simulink model "SchultzExample"  (R2017b)
settings: Solver=ode3  StartTime=0.0  StopTime=10.0  FixedStep=Ts  RelTol=1e-3
PreLoadFcn:
  | waijung.modelPreload; % Required for working with Waijung Blockset. Do not remove.
undefined symbols (not defined in the file): FiO2, HCLK, HSEOSC, Link, LQFP100, ST, STM32F407VG, STM32F4DISCOVERY, Ts
libraries: stm32f4_i2c_lib x17, simulink x3, stm32f4_io_lib x1, stm32f4_device_config_lib x1
(part 2 of 2)

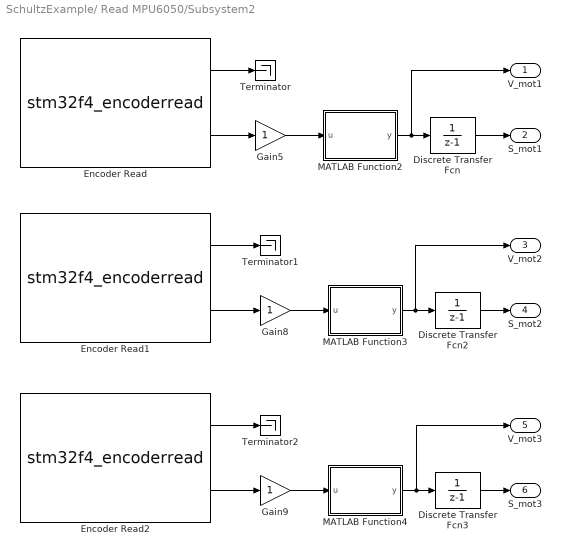
== system SchultzExample/ Read MPU6050/Subsystem2 ==
  Discrete Transfer Fcn : DiscreteTransferFcn  Denominator=[1 -1]
  Discrete Transfer Fcn2 : DiscreteTransferFcn  Denominator=[1 -1]
  Discrete Transfer Fcn3 : DiscreteTransferFcn  Denominator=[1 -1]
  Encoder Read : S-Function  FunctionName=stm32f4_encoderread  Parameters=sampletime,sampletimestr,blockid,timer,apb,portstr,pinstr,pinmat,chmat,filterstr,filter,factor,rstcnt,ppr  SFunctionDeploymentMode=off  EnableBusSupport=off  mask(stm32f4_encoderread){timer=3, ch1=B4, ch2=B5, ppr=65536, rstcnt=on, filterstr=No filter; sampling is done at fDTS, sampletime=Ts, sampletimestr=-1, blockid=ReadMPU6050Subsystem2EncoderRead, absresetinput=off, portpinstr=B4,B5, portstr=["B"], pinstr=["GPIO_Pin_4 | GPIO_Pin_5"], pinmat=[2 4 5], chmat=[1  2], apb=1, filter=0, factor=4}
      mask prompts: ch1 "Channel A Input Pin"; ch2 "Channel B Input Pin"; ppr "PPR (Number of pulses generated per revolution)"; rstcnt "Reset counter after every counter read"; filterstr "Built-in Input Capture Filter"; sampletime "Sample time (sec)"; sampletimestr "Compiled sample time (sec) in string"; absresetinput "Enable absolute position reset input signal"; portpinstr "Port pin string"; portstr "Port string"; pinstr "Pin string"; pinmat "Pin matrix"; chmat "Channel order"; filter "Filter ID"
      mask help:
      | The output Direction (uint32) is the direction of rotation either 0 or 1.
      |
      | The output Position (count) (uint32) is the count of number of edges of the encoder output signals from either channel A and B. The decoder is set to count at every rising and falling edge of both channel A and B (4x) or (x2) for one channel. For example, if an encoder has 180 pulses per revolution (PPS) and two channels are selected, the maximum count is 720 per revolution (4x180 = 720), i.e. from 0 to 719.
      mask init:
      | stm32f4_encoderread_callback('init');
      mask Help: web(fullfile(waijungdocroot,'stm32f4_encoderread.htm'),'-browser')
      mask TypeOptions timer: 1 | 2 | 3 | 4 | 5 | 8
      mask Callback timer: stm32f4_encoderread_callback('timer');
      mask TypeOptions ch1: Not available - Do not use | A6 | C6 | B4
      mask Callback ch1: stm32f4_encoderread_callback('chA');
      mask TypeOptions ch2: Not available - Do not use | A7 | C7 | B5
      mask Callback ch2: stm32f4_encoderread_callback('chB');
      mask Callback ppr: stm32f4_encoderread_callback('ppr');
      mask Callback rstcnt: stm32f4_encoderread_callback('rstcnt');
      mask TypeOptions filterstr: No filter; sampling is done at fDTS | fSAMPLING=fCK_INT; N=2 | fSAMPLING=fCK_INT; N=4 | fSAMPLING=fCK_INT; N=8 | fSAMPLING=fDTS/2; N=6 | fSAMPLING=fDTS/2; N=8 | fSAMPLING=fDTS/4; N=6 | fSAMPLING=fDTS/4; N=8 | fSAMPLING=fDTS/8; N=6 | fSAMPLING=fDTS/8; N=8 | fSAMPLING=fDTS/16; N=5 | fSAMPLING=fDTS/16; N=6 | fSAMPLING=fDTS/16; N=8 | fSAMPLING=fDTS/32; N=5 | fSAMPLING=fDTS/32; N=6 | fSAMPLING=fDTS/32; N=8
      mask Callback filterstr: stm32f4_encoderread_callback('filterstr');
      mask Callback sampletimestr: stm32f4_encoderread_callback('sampletimestr');
      mask Callback blockid: stm32f4_encoderread_callback('blockid');
      mask Display: text(0.05, 0.5, 'Timer: 3\nInput pins [CH_A, CH_B]: [B4,B5]\nRST Counter: Yes\nTs (sec): -1','ver','middle','hor','left');port_label('output', 1, 'Direction');port_label('output', 2, 'Position (count)')
  Encoder Read1 : S-Function  FunctionName=stm32f4_encoderread  Parameters=sampletime,sampletimestr,blockid,timer,apb,portstr,pinstr,pinmat,chmat,filterstr,filter,factor,rstcnt,ppr  SFunctionDeploymentMode=off  EnableBusSupport=off  mask(stm32f4_encoderread){timer=1, ch1=E9, ch2=E11, ppr=65536, rstcnt=on, filterstr=No filter; sampling is done at fDTS, sampletime=Ts, sampletimestr=-1, blockid=ReadMPU6050Subsystem2EncoderRead1, absresetinput=off, portpinstr=E9,E11, portstr=["E"], pinstr=["GPIO_Pin_9 | GPIO_Pin_11"], pinmat=[2 9 11], chmat=[1  2], apb=2, filter=0, factor=4}
      mask prompts: ch1 "Channel A Input Pin"; ch2 "Channel B Input Pin"; ppr "PPR (Number of pulses generated per revolution)"; rstcnt "Reset counter after every counter read"; filterstr "Built-in Input Capture Filter"; sampletime "Sample time (sec)"; sampletimestr "Compiled sample time (sec) in string"; absresetinput "Enable absolute position reset input signal"; portpinstr "Port pin string"; portstr "Port string"; pinstr "Pin string"; pinmat "Pin matrix"; chmat "Channel order"; filter "Filter ID"
      mask help:
      | The output Direction (uint32) is the direction of rotation either 0 or 1.
      |
      | The output Position (count) (uint32) is the count of number of edges of the encoder output signals from either channel A and B. The decoder is set to count at every rising and falling edge of both channel A and B (4x) or (x2) for one channel. For example, if an encoder has 180 pulses per revolution (PPS) and two channels are selected, the maximum count is 720 per revolution (4x180 = 720), i.e. from 0 to 719.
      mask init:
      | stm32f4_encoderread_callback('init');
      mask Help: web(fullfile(waijungdocroot,'stm32f4_encoderread.htm'),'-browser')
      mask TypeOptions timer: 1 | 2 | 3 | 4 | 5 | 8
      mask Callback timer: stm32f4_encoderread_callback('timer');
      mask TypeOptions ch1: Not available - Do not use | E9 | A8
      mask Callback ch1: stm32f4_encoderread_callback('chA');
      mask TypeOptions ch2: Not available - Do not use | E11 | A9
      mask Callback ch2: stm32f4_encoderread_callback('chB');
      mask Callback ppr: stm32f4_encoderread_callback('ppr');
      mask Callback rstcnt: stm32f4_encoderread_callback('rstcnt');
      mask TypeOptions filterstr: No filter; sampling is done at fDTS | fSAMPLING=fCK_INT; N=2 | fSAMPLING=fCK_INT; N=4 | fSAMPLING=fCK_INT; N=8 | fSAMPLING=fDTS/2; N=6 | fSAMPLING=fDTS/2; N=8 | fSAMPLING=fDTS/4; N=6 | fSAMPLING=fDTS/4; N=8 | fSAMPLING=fDTS/8; N=6 | fSAMPLING=fDTS/8; N=8 | fSAMPLING=fDTS/16; N=5 | fSAMPLING=fDTS/16; N=6 | fSAMPLING=fDTS/16; N=8 | fSAMPLING=fDTS/32; N=5 | fSAMPLING=fDTS/32; N=6 | fSAMPLING=fDTS/32; N=8
      mask Callback filterstr: stm32f4_encoderread_callback('filterstr');
      mask Callback sampletimestr: stm32f4_encoderread_callback('sampletimestr');
      mask Callback blockid: stm32f4_encoderread_callback('blockid');
      mask Display: text(0.05, 0.5, 'Timer: 1\nInput pins [CH_A, CH_B]: [E9,E11]\nRST Counter: Yes\nTs (sec): -1','ver','middle','hor','left');port_label('output', 1, 'Direction');port_label('output', 2, 'Position (count)')
  Encoder Read2 : S-Function  FunctionName=stm32f4_encoderread  Parameters=sampletime,sampletimestr,blockid,timer,apb,portstr,pinstr,pinmat,chmat,filterstr,filter,factor,rstcnt,ppr  SFunctionDeploymentMode=off  EnableBusSupport=off  mask(stm32f4_encoderread){timer=8, ch1=C6, ch2=C7, ppr=65536, rstcnt=on, filterstr=No filter; sampling is done at fDTS, sampletime=Ts, sampletimestr=-1, blockid=ReadMPU6050Subsystem2EncoderRead2, absresetinput=off, portpinstr=C6,C7, portstr=["C"], pinstr=["GPIO_Pin_6 | GPIO_Pin_7"], pinmat=[2 6 7], chmat=[1  2], apb=2, filter=0, factor=4}
      mask prompts: ch1 "Channel A Input Pin"; ch2 "Channel B Input Pin"; ppr "PPR (Number of pulses generated per revolution)"; rstcnt "Reset counter after every counter read"; filterstr "Built-in Input Capture Filter"; sampletime "Sample time (sec)"; sampletimestr "Compiled sample time (sec) in string"; absresetinput "Enable absolute position reset input signal"; portpinstr "Port pin string"; portstr "Port string"; pinstr "Pin string"; pinmat "Pin matrix"; chmat "Channel order"; filter "Filter ID"
      mask help:
      | The output Direction (uint32) is the direction of rotation either 0 or 1.
      |
      | The output Position (count) (uint32) is the count of number of edges of the encoder output signals from either channel A and B. The decoder is set to count at every rising and falling edge of both channel A and B (4x) or (x2) for one channel. For example, if an encoder has 180 pulses per revolution (PPS) and two channels are selected, the maximum count is 720 per revolution (4x180 = 720), i.e. from 0 to 719.
      mask init:
      | stm32f4_encoderread_callback('init');
      mask Help: web(fullfile(waijungdocroot,'stm32f4_encoderread.htm'),'-browser')
      mask TypeOptions timer: 1 | 2 | 3 | 4 | 5 | 8
      mask Callback timer: stm32f4_encoderread_callback('timer');
      mask TypeOptions ch1: Not available - Do not use | A6 | C6 | B4
      mask Callback ch1: stm32f4_encoderread_callback('chA');
      mask TypeOptions ch2: Not available - Do not use | A7 | C7 | B5
      mask Callback ch2: stm32f4_encoderread_callback('chB');
      mask Callback ppr: stm32f4_encoderread_callback('ppr');
      mask Callback rstcnt: stm32f4_encoderread_callback('rstcnt');
      mask TypeOptions filterstr: No filter; sampling is done at fDTS | fSAMPLING=fCK_INT; N=2 | fSAMPLING=fCK_INT; N=4 | fSAMPLING=fCK_INT; N=8 | fSAMPLING=fDTS/2; N=6 | fSAMPLING=fDTS/2; N=8 | fSAMPLING=fDTS/4; N=6 | fSAMPLING=fDTS/4; N=8 | fSAMPLING=fDTS/8; N=6 | fSAMPLING=fDTS/8; N=8 | fSAMPLING=fDTS/16; N=5 | fSAMPLING=fDTS/16; N=6 | fSAMPLING=fDTS/16; N=8 | fSAMPLING=fDTS/32; N=5 | fSAMPLING=fDTS/32; N=6 | fSAMPLING=fDTS/32; N=8
      mask Callback filterstr: stm32f4_encoderread_callback('filterstr');
      mask Callback sampletimestr: stm32f4_encoderread_callback('sampletimestr');
      mask Callback blockid: stm32f4_encoderread_callback('blockid');
      mask Display: text(0.05, 0.5, 'Timer: 8\nInput pins [CH_A, CH_B]: [C6,C7]\nRST Counter: Yes\nTs (sec): -1','ver','middle','hor','left');port_label('output', 1, 'Direction');port_label('output', 2, 'Position (count)')
  Gain5 : Gain  OutDataTypeStr=double
  Gain8 : Gain  OutDataTypeStr=double
  Gain9 : Gain  OutDataTypeStr=double
  MATLAB Function2 : MATLAB Function  TreatAsAtomicUnit=on
  MATLAB Function3 : MATLAB Function  TreatAsAtomicUnit=on
  MATLAB Function4 : MATLAB Function  TreatAsAtomicUnit=on
  Terminator : Terminator
  Terminator1 : Terminator
  Terminator2 : Terminator
  V_mot1 : Outport
  S_mot1 : Outport  Port=2
  V_mot2 : Outport  Port=3
  S_mot2 : Outport  Port=4
  V_mot3 : Outport  Port=5
  S_mot3 : Outport  Port=6
  wires:
  Encoder Read2/1 -> Terminator2/1
  Encoder Read1/1 -> Terminator1/1
  Encoder Read/1 -> Terminator/1
  Discrete Transfer Fcn/1 -> S_mot1/1
  Discrete Transfer Fcn2/1 -> S_mot2/1
  Discrete Transfer Fcn3/1 -> S_mot3/1
  Encoder Read2/2 -> Gain9/1
  MATLAB Function4/1(y) -> Discrete Transfer Fcn3/1, V_mot3/1
  Gain9/1 -> MATLAB Function4/1(u)
  Encoder Read1/2 -> Gain8/1
  MATLAB Function3/1(y) -> Discrete Transfer Fcn2/1, V_mot2/1
  Gain8/1 -> MATLAB Function3/1(u)
  MATLAB Function2/1(y) -> Discrete Transfer Fcn/1, V_mot1/1
  Encoder Read/2 -> Gain5/1
  Gain5/1 -> MATLAB Function2/1(u)

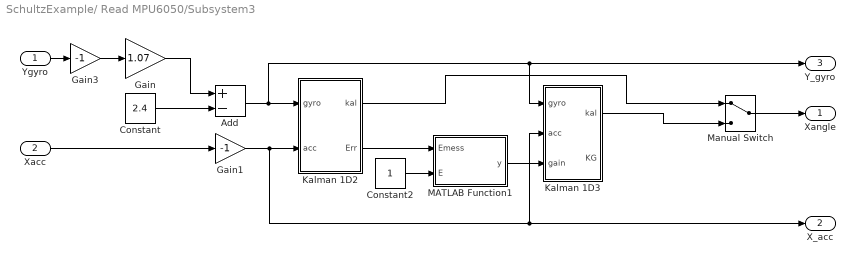
== system SchultzExample/ Read MPU6050/Subsystem3 ==
  Ygyro : Inport
  Xacc : Inport  Port=2
  Add : Sum  Inputs=+-
  Constant : Constant  Value=2.4
  Constant2 : Constant
  Gain : Gain  Gain=1.07
  Gain1 : Gain  Gain=-1  OutDataTypeStr=double
  Gain3 : Gain  Gain=-1  OutDataTypeStr=double
  Kalman 1D2 : Subsystem
  Kalman 1D3 : Subsystem
  MATLAB Function1 : MATLAB Function  TreatAsAtomicUnit=on
  Manual Switch : ManualSwitch
  Xangle : Outport
  X_acc : Outport  Port=2
  Y_gyro : Outport  Port=3
  wires:
  Constant/1 -> Add/2
  Gain/1 -> Add/1
  Gain3/1 -> Gain/1
  Add/1 -> Kalman 1D2/1(gyro), Y_gyro/1, Kalman 1D3/1(gyro)
  Gain1/1 -> Kalman 1D2/2(acc), Kalman 1D3/2(acc), X_acc/1
  MATLAB Function1/1(y) -> Kalman 1D3/3(gain)
  Kalman 1D2/2(Err) -> MATLAB Function1/1(Emess)
  Constant2/1 -> MATLAB Function1/2(E)
  Xacc/1 -> Gain1/1
  Ygyro/1 -> Gain3/1
  Manual Switch/1 -> Xangle/1
  Kalman 1D2/1(kal) -> Manual Switch/1
  Kalman 1D3/1(kal) -> Manual Switch/2

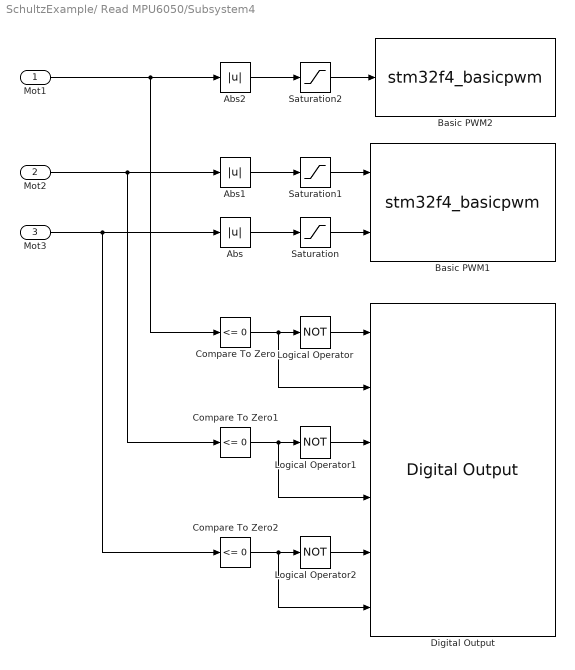
== system SchultzExample/ Read MPU6050/Subsystem4 ==
  Mot1 : Inport
  Mot2 : Inport  Port=2
  Mot3 : Inport  Port=3
  Abs : Abs
  Abs1 : Abs
  Abs2 : Abs
  Basic PWM1 : S-Function  FunctionName=stm32f4_basicpwm  Parameters=timer,pwmperiod,ch1pin,ch2pin,ch3pin,ch4pin,sampletime,sampletimestr,blockid,apb,portstr,pinstr,pinmat,timarr,timprescale,chmat,polaritystr  SFunctionDeploymentMode=off  EnableBusSupport=off  mask(stm32f4_basicpwm){timer=9, pwmperiod=50e-6, polarity=Active High, polaritystr=TIM_OCPolarity_High, ch1pin=A2, ch2pin=E6, ch3pin=Not available - Do not use, ch4pin=Not available - Do not use, sampletime=Ts, sampletimestr=-1, blockid=ReadMPU6050Subsystem4BasicPWM1, portpinstr=A2,E6,,, enablecustomportlabel=off, cinputportlabel=In1, In2, In3, In4, coutputportlabel=0, apb=2, portstr=["A","E"], pinstr=["GPIO_Pin_2","GPIO_Pin_6"], pinmat=[1 2;1 6], timarr=8399, timprescale=0, chmat=[1  2]}
      mask prompts: pwmperiod "PWM Period (seconds)"; ch1pin "Channel 1"; ch2pin "Channel 2"; ch3pin "Channel 3"; ch4pin "Channel 4"; sampletime "Sample time (sec)"; sampletimestr "Compiled sample time (sec) in string"; portpinstr "Port pin string"; enablecustomportlabel "Enable custom port labels"; cinputportlabel "Custom input port labels (Ex. In1, In2, In3)"; coutputportlabel "Custom output port labels (Ex. Out1, Out2, Out3)"; portstr "Port string"; pinstr "Pin string"; pinmat "Pin matrix"; timarr "Timer ARR"; timprescale "Timer PRESCALE"; chmat "Channel order"
      mask help:
      | This block implements basic Edge-aligned Pulse Width Modulation (PWM) generation.
      | All timers are 16-bit. The PWM period is fixed (per timer).
      mask init:
      | stm32f4_basicpwm_callback('init');
      mask Help: web(fullfile(waijungdocroot,'stm32f4_basicpwm.htm'),'-browser')
      mask TypeOptions timer: 1 | 2 | 3 | 4 | 5 | 8 | 9 | 10 | 11 | 12 | 13 | 14
      mask Callback timer: stm32f4_basicpwm_callback('timer');
      mask Callback pwmperiod: stm32f4_basicpwm_callback('pwmperiod');
      mask TypeOptions polarity: Active High | Active Low
      mask Callback polarity: stm32f4_basicpwm_callback('polarity');
      mask TypeOptions ch1pin: Not available - Do not use | E5 | A2
      mask Callback ch1pin: stm32f4_basicpwm_callback('ch1pin');
      mask TypeOptions ch2pin: Not available - Do not use | E6 | A3
      mask Callback ch2pin: stm32f4_basicpwm_callback('ch2pin');
      mask TypeOptions ch3pin: Not available - Do not use
      mask Callback ch3pin: stm32f4_basicpwm_callback('ch3pin');
      mask TypeOptions ch4pin: Not available - Do not use
      mask Callback ch4pin: stm32f4_basicpwm_callback('ch4pin');
      mask Callback sampletime: stm32f4_basicpwm_callback('sampletime');
      mask Callback sampletimestr: stm32f4_basicpwm_callback('sampletimestr');
      mask Callback blockid: stm32f4_basicpwm_callback('blockid');
      mask Callback enablecustomportlabel: stm32f4_basicpwm_callback('enablecustomportlabel');
      mask Display: text(0.95, 0.5, 'Timer: 9\nPolarity: Active High\nPeriod (sec) 50e-6\nTs (sec): -1','ver','middle','hor','right');port_label('input', 1,'CH1 (A2)');port_label('input', 2,'CH2 (E6)')
  Basic PWM2 : S-Function  FunctionName=stm32f4_basicpwm  Parameters=timer,pwmperiod,ch1pin,ch2pin,ch3pin,ch4pin,sampletime,sampletimestr,blockid,apb,portstr,pinstr,pinmat,timarr,timprescale,chmat,polaritystr  SFunctionDeploymentMode=off  EnableBusSupport=off  mask(stm32f4_basicpwm){timer=12, pwmperiod=50e-6, polarity=Active High, polaritystr=TIM_OCPolarity_High, ch1pin=B14, ch2pin=Not available - Do not use, ch3pin=Not available - Do not use, ch4pin=Not available - Do not use, sampletime=Ts, sampletimestr=-1, blockid=ReadMPU6050Subsystem4BasicPWM2, portpinstr=B14,,,, enablecustomportlabel=off, cinputportlabel=In1, In2, In3, In4, coutputportlabel=0, apb=1, portstr=["B"], pinstr=["GPIO_Pin_14"], pinmat=[1 14], timarr=4199, timprescale=0, chmat=[1]}
      mask prompts: pwmperiod "PWM Period (seconds)"; ch1pin "Channel 1"; ch2pin "Channel 2"; ch3pin "Channel 3"; ch4pin "Channel 4"; sampletime "Sample time (sec)"; sampletimestr "Compiled sample time (sec) in string"; portpinstr "Port pin string"; enablecustomportlabel "Enable custom port labels"; cinputportlabel "Custom input port labels (Ex. In1, In2, In3)"; coutputportlabel "Custom output port labels (Ex. Out1, Out2, Out3)"; portstr "Port string"; pinstr "Pin string"; pinmat "Pin matrix"; timarr "Timer ARR"; timprescale "Timer PRESCALE"; chmat "Channel order"
      mask help:
      | This block implements basic Edge-aligned Pulse Width Modulation (PWM) generation.
      | All timers are 16-bit. The PWM period is fixed (per timer).
      mask init:
      | stm32f4_basicpwm_callback('init');
      mask Help: web(fullfile(waijungdocroot,'stm32f4_basicpwm.htm'),'-browser')
      mask TypeOptions timer: 1 | 2 | 3 | 4 | 5 | 8 | 9 | 10 | 11 | 12 | 13 | 14
      mask Callback timer: stm32f4_basicpwm_callback('timer');
      mask Callback pwmperiod: stm32f4_basicpwm_callback('pwmperiod');
      mask TypeOptions polarity: Active High | Active Low
      mask Callback polarity: stm32f4_basicpwm_callback('polarity');
      mask TypeOptions ch1pin: Not available - Do not use | B14
      mask Callback ch1pin: stm32f4_basicpwm_callback('ch1pin');
      mask TypeOptions ch2pin: Not available - Do not use | B15
      mask Callback ch2pin: stm32f4_basicpwm_callback('ch2pin');
      mask TypeOptions ch3pin: Not available - Do not use
      mask Callback ch3pin: stm32f4_basicpwm_callback('ch3pin');
      mask TypeOptions ch4pin: Not available - Do not use
      mask Callback ch4pin: stm32f4_basicpwm_callback('ch4pin');
      mask Callback sampletime: stm32f4_basicpwm_callback('sampletime');
      mask Callback sampletimestr: stm32f4_basicpwm_callback('sampletimestr');
      mask Callback blockid: stm32f4_basicpwm_callback('blockid');
      mask Callback enablecustomportlabel: stm32f4_basicpwm_callback('enablecustomportlabel');
      mask Display: text(0.95, 0.5, 'Timer: 12\nPolarity: Active High\nPeriod (sec) 50e-6\nTs (sec): -1','ver','middle','hor','right');port_label('input', 1,'CH1 (B14)')
  Compare To Zero : simulink/Logic and Bit Operations/Compare To Zero  relop=<=  OutDataTypeStr=boolean
  Compare To Zero1 : simulink/Logic and Bit Operations/Compare To Zero  relop=<=  OutDataTypeStr=boolean
  Compare To Zero2 : simulink/Logic and Bit Operations/Compare To Zero  relop=<=  OutDataTypeStr=boolean
  Digital Output : stm32f4_io_lib/Digital Output  use_bitband=on  port=D  speed=100  porttype=Push Pull  porttypestr=PP  use_pin0=off  use_pin1=on  use_pin2=on  use_pin3=on  use_pin4=on  use_pin5=on  use_pin6=on  use_pin7=off  use_pin8=off  use_pin9=off  use_pin10=off  use_pin11=off  use_pin12=off  use_pin13=off  use_pin14=off  use_pin15=off  pinstr=GPIO_Pin_1 | GPIO_Pin_2 | GPIO_Pin_3 | GPIO_Pin_4 | GPIO_Pin_5 | GPIO_Pin_6  usedpinarray="[0  1  1  1  1  1  1  0  0  0  0  0  0  0  0  0]"  bitbandingstr=|  sampletime=Ts  sampletimestr=-1  blockid=ReadMPU6050Subsystem4DigitalOutput  enablecustomportlabel=off  globalinit=off  cinputportlabel=In1, In2  coutputportlabel=0
      | #define ReadMPU6050Subsystem4DigitalOutput_D1 Peripheral_BB(GPIOD->ODR, 1)  /* Output pin */
      | #define ReadMPU6050Subsystem4DigitalOutput_D2 Peripheral_BB(GPIOD->ODR, 2)  /* Output pin */
      | #define ReadMPU6050Subsystem4DigitalOutput_D3 Peripheral_BB(GPIOD->ODR, 3)  /* Output pin */
      | #define ReadMPU6050Subsystem4DigitalOutput_D4 Peripheral_BB(GPIOD->ODR, 4)  /* Output pin */
      | #define ReadMPU6050Subsystem4DigitalOutput_D5 Peripheral_BB(GPIOD->ODR, 5)  /* Output pin */
      | #define ReadMPU6050Subsystem4DigitalOutput_D6 Peripheral_BB(GPIOD->ODR, 6)  /* Output pin */
  Logical Operator : Logic  Operator=NOT  AllPortsSameDT=off  OutDataTypeStr=boolean
  Logical Operator1 : Logic  Operator=NOT  AllPortsSameDT=off  OutDataTypeStr=boolean
  Logical Operator2 : Logic  Operator=NOT  AllPortsSameDT=off  OutDataTypeStr=boolean
  Saturation : Saturate  UpperLimit=100  LowerLimit=0
  Saturation1 : Saturate  UpperLimit=100  LowerLimit=0
  Saturation2 : Saturate  UpperLimit=100  LowerLimit=0
  wires:
  Logical Operator1/1 -> Digital Output/3
  Saturation1/1 -> Basic PWM1/1
  Mot1/1 -> Abs2/1, Compare To Zero/1
  Abs2/1 -> Saturation2/1
  Compare To Zero1/1 -> Digital Output/4, Logical Operator1/1
  Logical Operator/1 -> Digital Output/1
  Compare To Zero/1 -> Digital Output/2, Logical Operator/1
  Abs/1 -> Saturation/1
  Mot3/1 -> Abs/1, Compare To Zero2/1
  Mot2/1 -> Abs1/1, Compare To Zero1/1
  Abs1/1 -> Saturation1/1
  Saturation2/1 -> Basic PWM2/1
  Saturation/1 -> Basic PWM1/2
  Compare To Zero2/1 -> Digital Output/6, Logical Operator2/1
  Logical Operator2/1 -> Digital Output/5

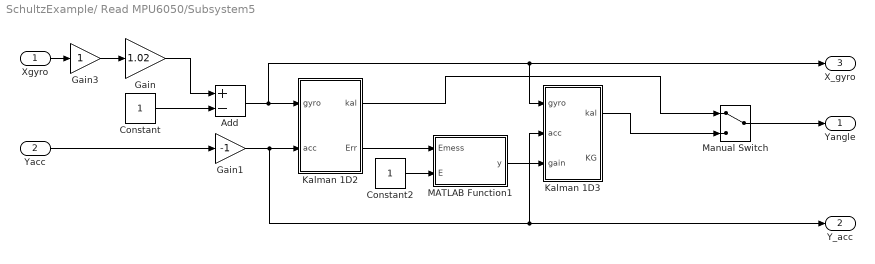
== system SchultzExample/ Read MPU6050/Subsystem5 ==
  Xgyro : Inport
  Yacc : Inport  Port=2
  Add : Sum  Inputs=+-
  Constant : Constant
  Constant2 : Constant
  Gain : Gain  Gain=1.02
  Gain1 : Gain  Gain=-1  OutDataTypeStr=double
  Gain3 : Gain  OutDataTypeStr=double
  Kalman 1D2 : Subsystem
  Kalman 1D3 : Subsystem
  MATLAB Function1 : MATLAB Function  TreatAsAtomicUnit=on
  Manual Switch : ManualSwitch
  Yangle : Outport
  Y_acc : Outport  Port=2
  X_gyro : Outport  Port=3
  wires:
  Xgyro/1 -> Gain3/1
  Yacc/1 -> Gain1/1
  Constant2/1 -> MATLAB Function1/2(E)
  Kalman 1D2/2(Err) -> MATLAB Function1/1(Emess)
  MATLAB Function1/1(y) -> Kalman 1D3/3(gain)
  Gain1/1 -> Y_acc/1, Kalman 1D3/2(acc), Kalman 1D2/2(acc)
  Add/1 -> Kalman 1D3/1(gyro), X_gyro/1, Kalman 1D2/1(gyro)
  Gain3/1 -> Gain/1
  Gain/1 -> Add/1
  Constant/1 -> Add/2
  Manual Switch/1 -> Yangle/1
  Kalman 1D2/1(kal) -> Manual Switch/1
  Kalman 1D3/1(kal) -> Manual Switch/2

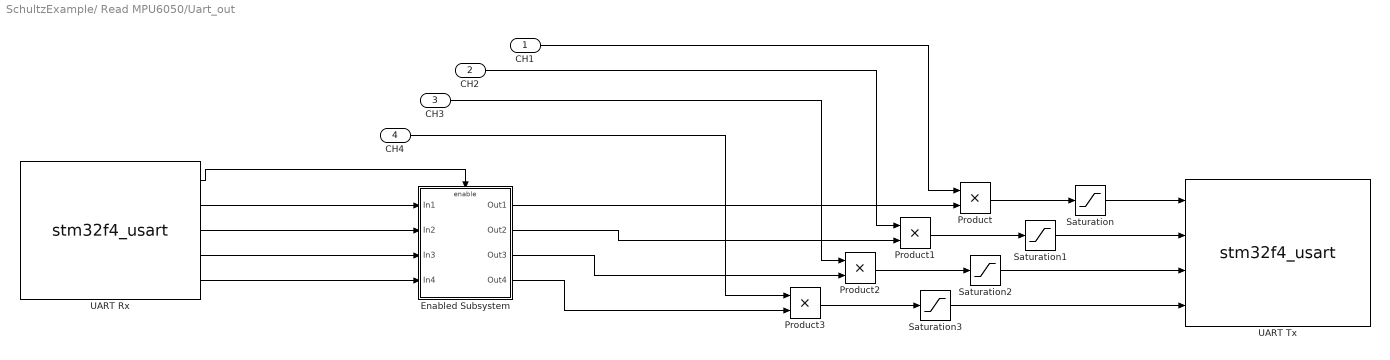
== system SchultzExample/ Read MPU6050/Uart_out ==
  CH1 : Inport
  CH2 : Inport  Port=2
  CH3 : Inport  Port=3
  CH4 : Inport  Port=4
  Enabled Subsystem : Subsystem  TreatAsAtomicUnit=on
  Product{,1..3} (4 alike) : Product
  Saturation{,1..3} (4 alike) : Saturate  UpperLimit=127  LowerLimit=-127  OutDataTypeStr=int8
  UART Rx : S-Function  Priority=1  FunctionName=stm32f4_usart  Parameters=configuration,uartmodule,transfer,baudrate,inputtype,outputtype,confstr,binheaderarray,binterminatorarray,asciiheader,asciiterminator,bindatalength,packetmode,varname,sampletime,sampletimestr,blockid  SFunctionDeploymentMode=off  EnableBusSupport=off  mask(stm32f4_usart){configuration=Rx, uartmodule=4, baudrate=115200, databits=8, parity=No, stopbit=1, remaptxpin=Not used, remaprxpin=Not used, flowcontrol=None, remapctspin=Not used, remaprtspin=Not used, advanceoptions=off, rxbuffersize=512, txbuffersize=512, transfer=Non-Blocking, packetmode=Binary, binheader='7E 7E', binterminator='03 03', porttype_double=0, porttype_single=0, porttype_int8=0, porttype_uint8=4, porttype_int16=0, porttype_uint16=0, porttype_int32=0, porttype_uint32=0, asciiformat='value=%d,%f', rx_asciiterminator=CRLF (0x0D 0x0A - "\r\n"), tx_asciiterminator=LF (0x0A - "\n"), storagename=<empty>, varname=, inputtype=[0], outputtype=[5 3  3 3 3 3], binheaderarray=[2 126  126], binterminatorarray=[2 3  3], bindatalength=4, asciiheader='value=%d,%f\r\n', asciiterminator=[2 13 10], sampletime=Ts, sampletimestr=-1, blockid=ReadMPU6050Uart_outUARTRx, confstr=[ "dummy", "0", "*", "*", "0", "*", "*", "0", "*", "*", "0", "*", "*", "1", "4", "4", "1", "4", "2", "512", "512", "1", "4", "115200", "8", "No", "1", "None", "UART4"], lastmodule=1}
      mask prompts: uartmodule "UART Module"; baudrate "Baud rate (bps)"; databits "Data bits"; stopbit "Stop bit"; remaptxpin "Tx Pin"; remaprxpin "Rx Pin"; flowcontrol "Hardware flow control"; remapctspin "HW Flow control, CTS Pin"; remaprtspin "HW Flow control, RTS Pin"; advanceoptions "Advance options"; rxbuffersize "Rx buffer size (bytes)"; txbuffersize "Tx buffer size (bytes)"; packetmode "Packet mode"; binheader "Binary header (example: '7E 7E')"; binterminator "Binary terminator (example: '03 03')"; porttype_double "Number of data port, type DOUBLE"; porttype_single "Number of data port, type SINGLE"; porttype_int8 "Number of data port, type INT8"; porttype_uint8 "Number of data port, type UINT8"; porttype_int16 "Number of data port, type INT16"; porttype_uint16 "Number of data port, type UINT16"; porttype_int32 "Number of data port, type INT32"; porttype_uint32 "Number of data port, type UINT32"; asciiformat "Ascii format"; rx_asciiterminator "End of packet"; tx_asciiterminator "End of packet"; storagename "Buffer"; varname "Var name"; inputtype "Input data type"; outputtype "Output data type"; binheaderarray "Binary header"; binterminatorarray "Binary terminator"; bindatalength "Binary data length"; asciiheader "Ascii header (printf format)"; asciiterminator "Ascii terminator"; sampletime "Sample time (sec)"; sampletimestr "Compiled sample time (sec) in string"; confstr "Configuration string"; lastmodule "Last module selected"
      mask help:
      | Data type for Ascii format
      | %u, %i, %d, %o, %x: uint32
      | %e, %g, %f: single
      | %c: int8
      mask init:
      | stm32f4_usart_callback('init');
      mask Help: web(fullfile(waijungdocroot,'stm32f4_usart_rx.htm'), '-browser')
      mask TypeOptions configuration: Setup | Tx | Rx
      mask Callback configuration: stm32f4_usart_callback('configuration');
      mask TypeOptions uartmodule: 1 | 2 | 3 | 4 | 5 | 6
      mask Callback uartmodule: stm32f4_usart_callback('uartmodule');
      mask Callback baudrate: stm32f4_usart_callback('baudrate');
      mask TypeOptions databits: 8
      mask TypeOptions parity: No | Odd | Even
      mask TypeOptions stopbit: 0.5 | 1 | 1.5 | 2
      mask TypeOptions remaptxpin: Not used | A9 | B6
      mask TypeOptions remaprxpin: Not used | A10 | B7
      mask TypeOptions flowcontrol: None | RTS | CTS | RTS/CTS
      mask Callback flowcontrol: stm32f4_usart_callback('flowcontrol');
      mask TypeOptions remapctspin: Not used | A11
      mask TypeOptions remaprtspin: Not used | A12
      mask Callback advanceoptions: stm32f4_usart_callback('advanceoptions');
      mask TypeOptions rxbuffersize: 16 | 32 | 64 | 128 | 256 | 512 | 1024 | 2048
      mask TypeOptions txbuffersize: 16 | 32 | 64 | 128 | 256 | 512 | 1024 | 2048
      mask TypeOptions transfer: Blocking | Non-Blocking
      mask Callback transfer: stm32f4_usart_callback('transfer');
      mask TypeOptions packetmode: Ascii | Binary | Binary Vector | String Buffer | Raw Buffer
      mask Callback packetmode: stm32f4_usart_callback('packetmode');
      mask Callback binheader: stm32f4_usart_callback('binheader');
      mask Callback binterminator: stm32f4_usart_callback('binterminator');
      mask Callback porttype_double: stm32f4_usart_callback('porttype');
      mask Callback porttype_single: stm32f4_usart_callback('porttype');
      mask Callback porttype_int8: stm32f4_usart_callback('porttype');
      mask Callback porttype_uint8: stm32f4_usart_callback('porttype');
      mask Callback porttype_int16: stm32f4_usart_callback('porttype');
      mask Callback porttype_uint16: stm32f4_usart_callback('porttype');
      mask Callback porttype_int32: stm32f4_usart_callback('porttype');
      mask Callback porttype_uint32: stm32f4_usart_callback('porttype');
      mask Callback asciiformat: stm32f4_usart_callback('asciiformat');
      mask TypeOptions rx_asciiterminator: CR (0x0D - "\r") | LF (0x0A - "\n") | CRLF (0x0D 0x0A - "\r\n")
      mask Callback rx_asciiterminator: stm32f4_usart_callback('rx_asciiterminator');
      mask TypeOptions tx_asciiterminator: CR (0x0D - "\r") | LF (0x0A - "\n") | CRLF (0x0D 0x0A - "\r\n") | None
      mask Callback tx_asciiterminator: stm32f4_usart_callback('tx_asciiterminator');
      mask TypeOptions storagename: <empty>
      mask Callback storagename: stm32f4_usart_callback('storagename');
      mask Callback varname: stm32f4_usart_callback('varname');
      mask Callback sampletime: stm32f4_usart_callback('sampletime');
      mask Callback sampletimestr: stm32f4_usart_callback('sampletimestr');
      mask Callback blockid: stm32f4_usart_callback('blockid');
      mask Display: text(0.05, 0.5, 'Module: UART4_Rx\nPacket: Binary\nTransfer: Non-Blocking\nTs (sec): -1','ver','middle','hor','left'); port_label('output', 1,'READY'); port_label('output', 2,'uint8'); port_label('output', 3,'uint8'); port_label('output', 4,'uint8'); port_label('output', 5,'uint8');
  UART Tx : S-Function  Priority=1  FunctionName=stm32f4_usart  Parameters=configuration,uartmodule,transfer,baudrate,inputtype,outputtype,confstr,binheaderarray,binterminatorarray,asciiheader,asciiterminator,bindatalength,packetmode,varname,sampletime,sampletimestr,blockid  SFunctionDeploymentMode=off  EnableBusSupport=off  mask(stm32f4_usart){configuration=Tx, uartmodule=4, baudrate=115200, databits=8, parity=No, stopbit=1, remaptxpin=Not used, remaprxpin=Not used, flowcontrol=None, remapctspin=Not used, remaprtspin=Not used, advanceoptions=off, rxbuffersize=512, txbuffersize=512, transfer=Non-Blocking, packetmode=Binary, binheader='', binterminator='', porttype_double=0, porttype_single=0, porttype_int8=4, porttype_uint8=0, porttype_int16=0, porttype_uint16=0, porttype_int32=0, porttype_uint32=0, asciiformat='value=%d,%f', rx_asciiterminator=CRLF (0x0D 0x0A - "\r\n"), tx_asciiterminator=CRLF (0x0D 0x0A - "\r\n"), storagename=<empty>, varname=, inputtype=[4  2 2 2 2], outputtype=[0], binheaderarray=[0 ], binterminatorarray=[0 ], bindatalength=4, asciiheader='value=%d,%f\r\n', asciiterminator=[2 13 10], sampletime=Ts, sampletimestr=-1, blockid=ReadMPU6050Uart_outUARTTx, confstr=[ "dummy", "0", "*", "*", "0", "*", "*", "0", "*", "*", "0", "*", "*", "1", "4", "4", "1", "4", "2", "512", "512", "1", "4", "115200", "8", "No", "1", "None", "UART4"], lastmodule=1}
      mask prompts: uartmodule "UART Module"; baudrate "Baud rate (bps)"; databits "Data bits"; stopbit "Stop bit"; remaptxpin "Tx Pin"; remaprxpin "Rx Pin"; flowcontrol "Hardware flow control"; remapctspin "HW Flow control, CTS Pin"; remaprtspin "HW Flow control, RTS Pin"; advanceoptions "Advance options"; rxbuffersize "Rx buffer size (bytes)"; txbuffersize "Tx buffer size (bytes)"; packetmode "Packet mode"; binheader "Binary header (example: '7E 7E')"; binterminator "Binary terminator (example: '03 03')"; porttype_double "Number of data port, type DOUBLE"; porttype_single "Number of data port, type SINGLE"; porttype_int8 "Number of data port, type INT8"; porttype_uint8 "Number of data port, type UINT8"; porttype_int16 "Number of data port, type INT16"; porttype_uint16 "Number of data port, type UINT16"; porttype_int32 "Number of data port, type INT32"; porttype_uint32 "Number of data port, type UINT32"; asciiformat "Ascii format"; rx_asciiterminator "End of packet"; tx_asciiterminator "End of packet"; storagename "Buffer"; varname "Var name"; inputtype "Input data type"; outputtype "Output data type"; binheaderarray "Binary header"; binterminatorarray "Binary terminator"; bindatalength "Binary data length"; asciiheader "Ascii header (printf format)"; asciiterminator "Ascii terminator"; sampletime "Sample time (sec)"; sampletimestr "Compiled sample time (sec) in string"; confstr "Configuration string"; lastmodule "Last module selected"
      mask help:
      | Data type for Ascii format
      | %u, %i, %d, %o, %x: uint32
      | %e, %g, %f: single
      | %c: int8
      mask init:
      | stm32f4_usart_callback('init');
      mask Help: web(fullfile(waijungdocroot,'stm32f4_usart_tx.htm'), '-browser')
      mask TypeOptions configuration: Setup | Tx | Rx
      mask Callback configuration: stm32f4_usart_callback('configuration');
      mask TypeOptions uartmodule: 1 | 2 | 3 | 4 | 5 | 6
      mask Callback uartmodule: stm32f4_usart_callback('uartmodule');
      mask Callback baudrate: stm32f4_usart_callback('baudrate');
      mask TypeOptions databits: 8
      mask TypeOptions parity: No | Odd | Even
      mask TypeOptions stopbit: 0.5 | 1 | 1.5 | 2
      mask TypeOptions remaptxpin: Not used | A9 | B6
      mask TypeOptions remaprxpin: Not used | A10 | B7
      mask TypeOptions flowcontrol: None | RTS | CTS | RTS/CTS
      mask Callback flowcontrol: stm32f4_usart_callback('flowcontrol');
      mask TypeOptions remapctspin: Not used | A11
      mask TypeOptions remaprtspin: Not used | A12
      mask Callback advanceoptions: stm32f4_usart_callback('advanceoptions');
      mask TypeOptions rxbuffersize: 16 | 32 | 64 | 128 | 256 | 512 | 1024 | 2048
      mask TypeOptions txbuffersize: 16 | 32 | 64 | 128 | 256 | 512 | 1024 | 2048
      mask TypeOptions transfer: Blocking | Non-Blocking
      mask Callback transfer: stm32f4_usart_callback('transfer');
      mask TypeOptions packetmode: Ascii | Binary | Binary Vector | String Buffer
      mask Callback packetmode: stm32f4_usart_callback('packetmode');
      mask Callback binheader: stm32f4_usart_callback('binheader');
      mask Callback binterminator: stm32f4_usart_callback('binterminator');
      mask Callback porttype_double: stm32f4_usart_callback('porttype');
      mask Callback porttype_single: stm32f4_usart_callback('porttype');
      mask Callback porttype_int8: stm32f4_usart_callback('porttype');
      mask Callback porttype_uint8: stm32f4_usart_callback('porttype');
      mask Callback porttype_int16: stm32f4_usart_callback('porttype');
      mask Callback porttype_uint16: stm32f4_usart_callback('porttype');
      mask Callback porttype_int32: stm32f4_usart_callback('porttype');
      mask Callback porttype_uint32: stm32f4_usart_callback('porttype');
      mask Callback asciiformat: stm32f4_usart_callback('asciiformat');
      mask TypeOptions rx_asciiterminator: CR (0x0D - "\r") | LF (0x0A - "\n") | CRLF (0x0D 0x0A - "\r\n")
      mask Callback rx_asciiterminator: stm32f4_usart_callback('rx_asciiterminator');
      mask TypeOptions tx_asciiterminator: CR (0x0D - "\r") | LF (0x0A - "\n") | CRLF (0x0D 0x0A - "\r\n") | None
      mask Callback tx_asciiterminator: stm32f4_usart_callback('tx_asciiterminator');
      mask TypeOptions storagename: <empty>
      mask Callback storagename: stm32f4_usart_callback('storagename');
      mask Callback varname: stm32f4_usart_callback('varname');
      mask Callback sampletime: stm32f4_usart_callback('sampletime');
      mask Callback sampletimestr: stm32f4_usart_callback('sampletimestr');
      mask Callback blockid: stm32f4_usart_callback('blockid');
      mask Display: text(0.5, 0.5, 'Module: UART4_Tx\nPacket: Binary\nTransfer: Non-Blocking\nTs (sec): -1','ver','middle','hor','center'); port_label('input', 1,'int8'); port_label('input', 2,'int8'); port_label('input', 3,'int8'); port_label('input', 4,'int8');
  wires:
  Enabled Subsystem/4(Out4) -> Product3/2
  Enabled Subsystem/3(Out3) -> Product2/2
  Enabled Subsystem/2(Out2) -> Product1/2
  Enabled Subsystem/1(Out1) -> Product/2
  UART Rx/5 -> Enabled Subsystem/4(In4)
  UART Rx/4 -> Enabled Subsystem/3(In3)
  UART Rx/3 -> Enabled Subsystem/2(In2)
  UART Rx/2 -> Enabled Subsystem/1(In1)
  CH4/1 -> Product3/1
  CH1/1 -> Product/1
  CH3/1 -> Product2/1
  CH2/1 -> Product1/1
  Product2/1 -> Saturation2/1
  Product1/1 -> Saturation1/1
  Product3/1 -> Saturation3/1
  Product/1 -> Saturation/1
  UART Rx/1 -> Enabled Subsystem/Enable
  Saturation/1 -> UART Tx/1
  Saturation1/1 -> UART Tx/2
  Saturation2/1 -> UART Tx/3
  Saturation3/1 -> UART Tx/4

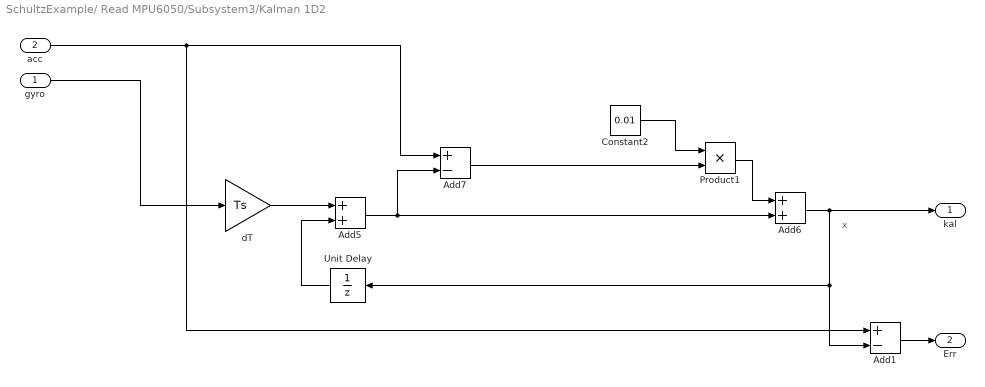
== system SchultzExample/ Read MPU6050/Subsystem3/Kalman 1D2 ==
  note: x
  gyro : Inport
  acc : Inport  Port=2
  Add1 : Sum  Inputs=+-
  Add5 : Sum
  Add6 : Sum
  Add7 : Sum  Inputs=+-
  Constant2 : Constant  Value=0.01
  Product1 : Product
  Unit Delay : UnitDelay  SampleTime=-1
  dT : Gain  Gain=Ts
  kal : Outport
  Err : Outport  Port=2
  wires:
  Constant2/1 -> Product1/1
  Add7/1 -> Product1/2
  Product1/1 -> Add6/1
  gyro/1 -> dT/1
  dT/1 -> Add5/1
  Add5/1 -> Add6/2, Add7/2
  Unit Delay/1 -> Add5/2
  Add6/1 -> Unit Delay/1, Add1/2, kal/1
  acc/1 -> Add7/1, Add1/1
  Add1/1 -> Err/1

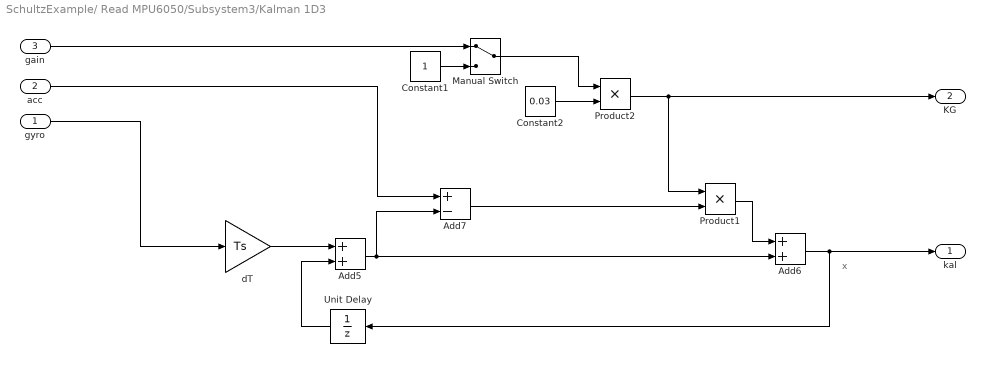
== system SchultzExample/ Read MPU6050/Subsystem3/Kalman 1D3 ==
  note: x
  gyro : Inport
  acc : Inport  Port=2
  gain : Inport  Port=3
  Add5 : Sum
  Add6 : Sum
  Add7 : Sum  Inputs=+-
  Constant1 : Constant
  Constant2 : Constant  Value=0.03
  Manual Switch : ManualSwitch
  Product1 : Product
  Product2 : Product
  Unit Delay : UnitDelay  SampleTime=-1
  dT : Gain  Gain=Ts
  kal : Outport
  KG : Outport  Port=2
  wires:
  Constant2/1 -> Product2/2
  Product2/1 -> KG/1, Product1/1
  acc/1 -> Add7/1
  Add6/1 -> kal/1, Unit Delay/1
  Unit Delay/1 -> Add5/2
  Add5/1 -> Add6/2, Add7/2
  dT/1 -> Add5/1
  gyro/1 -> dT/1
  Product1/1 -> Add6/1
  Add7/1 -> Product1/2
  gain/1 -> Manual Switch/1
  Manual Switch/1 -> Product2/1
  Constant1/1 -> Manual Switch/2

== system SchultzExample/ Read MPU6050/Subsystem5/Kalman 1D2 ==
  note: x
  gyro : Inport
  acc : Inport  Port=2
  Add1 : Sum  Inputs=+-
  Add5 : Sum
  Add6 : Sum
  Add7 : Sum  Inputs=+-
  Constant2 : Constant  Value=0.01
  Product1 : Product
  Unit Delay : UnitDelay  SampleTime=-1
  dT : Gain  Gain=Ts
  kal : Outport
  Err : Outport  Port=2
  wires:
  Add1/1 -> Err/1
  acc/1 -> Add1/1, Add7/1
  Add6/1 -> kal/1, Add1/2, Unit Delay/1
  Unit Delay/1 -> Add5/2
  Add5/1 -> Add7/2, Add6/2
  dT/1 -> Add5/1
  gyro/1 -> dT/1
  Product1/1 -> Add6/1
  Add7/1 -> Product1/2
  Constant2/1 -> Product1/1

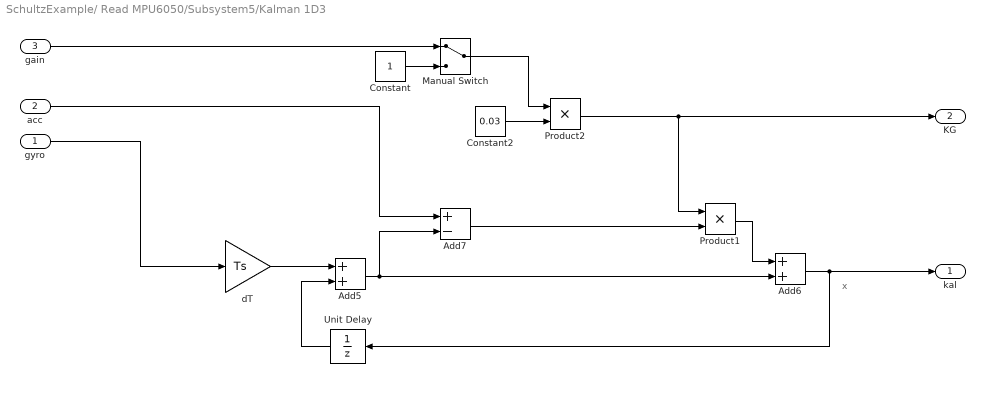
== system SchultzExample/ Read MPU6050/Subsystem5/Kalman 1D3 ==
  note: x
  gyro : Inport
  acc : Inport  Port=2
  gain : Inport  Port=3
  Add5 : Sum
  Add6 : Sum
  Add7 : Sum  Inputs=+-
  Constant : Constant
  Constant2 : Constant  Value=0.03
  Manual Switch : ManualSwitch
  Product1 : Product
  Product2 : Product
  Unit Delay : UnitDelay  SampleTime=-1
  dT : Gain  Gain=Ts
  kal : Outport
  KG : Outport  Port=2
  wires:
  Add7/1 -> Product1/2
  Product1/1 -> Add6/1
  gyro/1 -> dT/1
  dT/1 -> Add5/1
  Add5/1 -> Add6/2, Add7/2
  Unit Delay/1 -> Add5/2
  Add6/1 -> Unit Delay/1, kal/1
  acc/1 -> Add7/1
  Product2/1 -> Product1/1, KG/1
  Constant2/1 -> Product2/2
  Constant/1 -> Manual Switch/2
  Manual Switch/1 -> Product2/1
  gain/1 -> Manual Switch/1

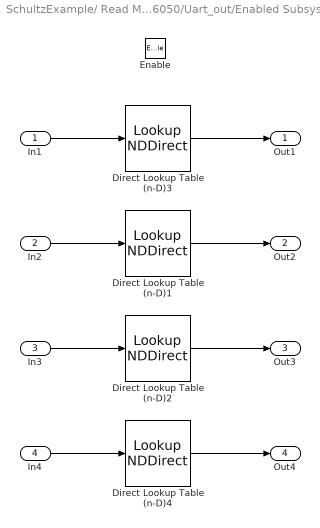
== system SchultzExample/ Read MPU6050/Uart_out/Enabled Subsystem ==
  In1 : Inport
  In2 : Inport  Port=2
  In3 : Inport  Port=3
  In4 : Inport  Port=4
  Enable : EnablePort
  Direct Lookup Table (n-D){1..4} (4 alike) : LookupNDDirect  NumberOfTableDimensions=1  Table=[0.001;0.002;0.005;0.01;0.02;0.05;0.1;0.2;0.5;1;2;5;10;20;50;100;200;500;1000]
  Out1 : Outport
  Out2 : Outport  Port=2
  Out3 : Outport  Port=3
  Out4 : Outport  Port=4
  wires:
  Direct Lookup Table (n-D)4/1 -> Out4/1
  Direct Lookup Table (n-D)2/1 -> Out3/1
  Direct Lookup Table (n-D)1/1 -> Out2/1
  In2/1 -> Direct Lookup Table (n-D)1/1
  In3/1 -> Direct Lookup Table (n-D)2/1
  In4/1 -> Direct Lookup Table (n-D)4/1
  Direct Lookup Table (n-D)3/1 -> Out1/1
  In1/1 -> Direct Lookup Table (n-D)3/1

== matlab function SchultzExample/ Read MPU6050/Subsystem3/MATLAB Function1 ==
  data: Emess input; y output; E input
function y = fcn(Emess,E)
%#codegen
s=abs(Emess);
y=E/(E+s);
if (y<0.1) y=0.1; end;

== matlab function SchultzExample/ Read MPU6050/Subsystem2/MATLAB Function2 ==
  data: u input; y output
function y = fcn(u)
%#codegen
y=u;
if (u>33000)
    y=y-65536;
end;

== matlab function SchultzExample/ Read MPU6050/Subsystem2/MATLAB Function3 ==
  data: u input; y output
function y = fcn(u)
%#codegen
y=u;
if (u>33000)
    y=y-65536;
end;

== matlab function SchultzExample/ Read MPU6050/Subsystem2/MATLAB Function4 ==
  data: u input; y output
function y = fcn(u)
%#codegen
y=u;
if (u>33000)
    y=y-65536;
end;

== matlab function SchultzExample/ Read MPU6050/Subsystem1/MATLAB Function1 ==
  data: Rx input; dir output; velo output; dir1 input; incd input; incv input; velo1 input
function [dir,velo] = fcn(Rx,dir1,incd,incv,velo1)
%#codegen
%r=114 l=108,u=117,d=100,n=110
dir=dir1; velo=velo1;
switch Rx         % r,l,u,d,n
    case 114
        dir=dir+incd;  
        if (dir>=100) dir=100; end      % r
    case 108
        dir=dir-incd;        % l
        if (dir<=-100) dir=-100; end      % r
    case 117
        velo=velo+incv;      % u
        if (velo>=100) velo=100; end      % r
    case 100
        velo=velo-incv;      % d
        if (velo<=-100) velo=-100; end      % r
    case 110    
        dir=0; velo=0;    % n
end

== matlab function SchultzExample/ Read MPU6050/Subsystem5/MATLAB Function1 ==
  data: Emess input; y output; E input
function y = fcn(Emess,E)
%#codegen
s=abs(Emess);
y=E/(E+s);
if (y<0.1) y=0.1; end;
